simulink model "fullrbdigeconverter"  (R2018b)
settings: Solver=FixedStepAuto  StartTime=0.0  StopTime=0.1  FixedStep=5e-6  RelTol=1e-3
libraries: powerlib x9, powerlib_meascontrol x1
settings Model: Creator=robom  LastModifiedBy=robom

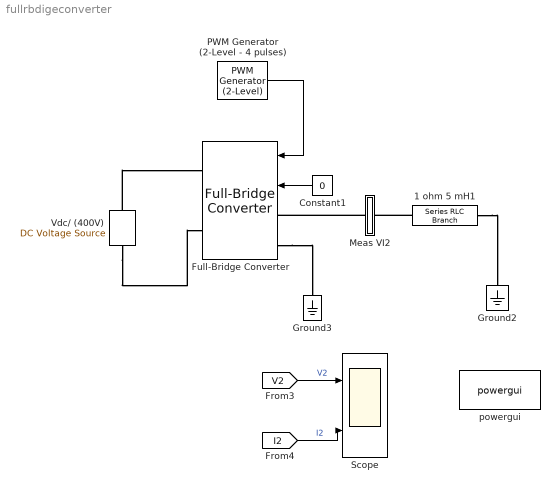
== system fullrbdigeconverter ==
  1 ohm 5 mH1 : powerlib/Elements/Series RLC Branch  LConnTagsString=__new0  RConnTagsString=__new0  BranchType=RL  Resistance=1  Inductance=5e-3  SetiL0=off  InitialCurrent=0  Capacitance=400e-6  Setx0=off  InitialVoltage=0  Measurements=None
      settings: SourceProductName=Simscape Electrical
  Constant1 : Constant  Value=0
  Full-Bridge Converter : powerlib/Power Electronics/Full-Bridge Converter  ModelType=Switching devices  Ron=1e-3  Rs=1e6  Cs=inf  Vforward=[0,0]  Ron_Diode=1e-3  Rs_Diode=1e6  Cs_Diode=inf  Vf_Diode=1e-3  Rs_CurrentSource=inf
      settings: SourceProductName=Simscape Electrical  SourceProductBaseCode=PS
  Ground2 : powerlib/Elements/Ground  LConnTagsString=a
      settings: SourceProductName=Simscape Electrical
  Ground3 : powerlib/Elements/Ground  LConnTagsString=a
      settings: SourceProductName=Simscape Electrical
  Meas VI2 : Subsystem
  PWM Generator (2-Level - 4 pulses) : powerlib_meascontrol/Pulse & Signal Generators/PWM Generator (2-Level)  ModulatorType=Single-phase full-bridge (4 pulses)  ModulatorMode=Unsynchronized  Fc=27*60  Pc=90  nF=27  MinMax="[ -1  1 ]"  SamplingTechnique=Natural  ModulatingSignals=off  m=0.8  Freq=60  Phase=0  Ts=5e-6  ShowCarrierOutport=off
  Scope : Scope  NumInputPorts=2
  Vdc/ (400V) : powerlib/Electrical Sources/DC Voltage Source  Amplitude=400  Measurements=None
      settings: SourceProductName=Simscape Electrical
  powergui : powerlib/powergui  Priority=1  SimulationMode=Discrete  SampleTime=5e-6  frequency=60  Iterations=50  frequencyindice=0  Pbase=100e6  ErrMax=1e-4  UnitsV=kV  UnitsW=MW  buscounter=0  FunctionMessages=off  echomessages=off  EnableUseOfTLC=off  CurrentSourceSwitches=off  DisableSnubberDevices=off  DisableRonSwitches=off  DisableVfSwitches=off  DisplayEquations=off  SolverType=Tustin/Backward Euler (TBE)  Interpol=off  ExternalGateDelay=off  methode=off  Ts=100  x0status=blocks  SPID=off  SwTol=0  HookPort=off  RestoreLinks=warning  ResistiveCurrentMeasurement=off  Frange=[0:2:500]  Ylog=off  Xlog=on  ShowGrid=off  save=off  variable=ZData  structure=ScopeDataForFFT  ZoomFFT=off  StartTime=0.07-2/60  cycles=2  DisplayStyle=1  fundamental=60  FreqAxis=off  MaxFrequency=5000  frequencyindicesteady=1  RmsSteady=1  display=off
      settings: SourceProductName=Simscape Electrical
  wires:
  [I2] -> Scope/2  "I2"
  [V2] -> Scope/1  "V2"
  PWM Generator (2-Level - 4 pulses)/1 -> Full-Bridge Converter/1
  Constant1/1 -> Full-Bridge Converter/2
  connections:
  Vdc/ (400V)/LConn1 -- Full-Bridge Converter/RConn2
  Full-Bridge Converter/LConn2 -- Ground3/LConn1
  Vdc/ (400V)/RConn1 -- Full-Bridge Converter/RConn1
  1 ohm 5 mH1/LConn1 -- Meas VI2/RConn1
  Meas VI2/LConn1 -- Full-Bridge Converter/LConn1
  1 ohm 5 mH1/RConn1 -- Ground2/LConn1

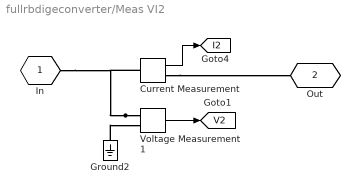
== system fullrbdigeconverter/Meas VI2 ==
  Current Measurement : powerlib/Measurements/Current Measurement  PhasorSimulation=off  OutputType=Complex  PSBequivalent=0
      settings: SourceProductName=Simscape Electrical
  Ground2 : powerlib/Elements/Ground  LConnTagsString=a
      settings: SourceProductName=Simscape Electrical
  Voltage Measurement1 : powerlib/Measurements/Voltage Measurement  Tag=PoWeRsYsTeMmEaSuReMeNt  PhasorSimulation=off  OutputType=Magnitude  PSBequivalent=0
      settings: SourceProductName=Simscape Electrical
  In : PMIOPort  Tag=PMCPort  Side=Left
  Out : PMIOPort  Tag=PMCPort  Port=2  Side=Right
  tag scope: I2=global, V2=global
  wires:
  Voltage Measurement1/1 -> [V2]
  Current Measurement/1 -> [I2]
  connections:
  Current Measurement/RConn1 -- Out/RConn1
  Voltage Measurement1/LConn1 -- Current Measurement/LConn1 -- In/RConn1
  Ground2/LConn1 -- Voltage Measurement1/LConn2
